simulink model "Copy_of_Single_Phase_SAPF_16apr"  (R2017a)
settings: Solver=ode45  StartTime=0.0  StopTime=10  RelTol=1e-3  EnableMultiTasking=on
libraries: powerlib x23, simulink x1
settings Model: Creator=Niranjan  LastModifiedBy=Dell
settings DataIOCC: LimitDataPoints=on  SaveFormat=Array
settings OptimizationCC: LifeSpan=inf
settings DebuggingCC: SolverPrmCheckMsg=warning  SFUnexpectedBacktrackingDiag=warning  SFNoUnconditionalDefaultTransitionDiag=warning  SFExecutionAtInitializationDiag=none
settings HardwareCC: ProdBitPerPointer=32  ProdBitPerSizeT=32  ProdBitPerPtrDiffT=32  ProdLargestAtomicFloat=None  ProdIntDivRoundTo=Undefined  ProdEndianess=Unspecified  ProdWordSize=32  ProdHWDeviceType=32-bit Generic
settings ModelReferenceCC: PropagateSignalLabelsOutOfModel=off
settings GRTTargetCC: TargetLangStandard=C89/C90 (ANSI)  GeneratePreprocessorConditionals=Disable all
settings ConfigComp: CovMetricSettings=dw  CovHtmlReporting=on  CovSaveCumulativeToWorkspaceVar=on  CovSaveSingleToWorkspaceVar=on  CovExternalEMLEnable=off  CovSFcnEnable=off

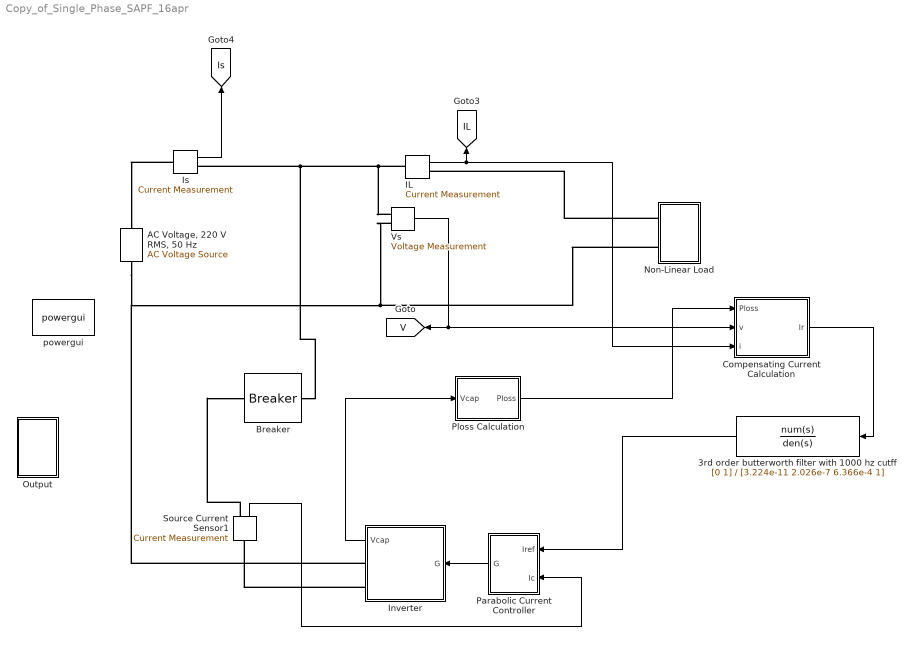
== system Copy_of_Single_Phase_SAPF_16apr ==
  3rd order butterworth filter with 1000 hz cutff : TransferFcn  Numerator=[0 1]  Denominator=[3.224e-11 2.026e-7 6.366e-4 1]
  "AC Voltage, 220 V RMS, 50 Hz" : powerlib/Electrical Sources/AC Voltage Source  Amplitude=311.13  Phase=0  Frequency=50  SampleTime=0  Measurements=None  BusType=swing  Pref=10e3  Qref=0  Qmin=-inf  Qmax=+inf
  Breaker : powerlib/Elements/Breaker  InitialState=0  SwitchingTimes=[0.965]  External=off  BreakerResistance=0.01  SnubberResistance=1e6  SnubberCapacitance=inf  Measurements=None  MoreParameters=on  NoBreakLoop=off
      settings: SourceProductName=Simscape Power Systems
  Compensating Current Calculation : Subsystem
  IL : powerlib/Measurements/Current Measurement  PhasorSimulation=off  OutputType=Complex  PSBequivalent=0
  Inverter : Subsystem
  Is : powerlib/Measurements/Current Measurement  PhasorSimulation=off  OutputType=Complex  PSBequivalent=0
  Non-Linear Load : Subsystem
  Output : Subsystem
  Parabolic Current Controller : Subsystem
  Ploss Calculation : Subsystem
  Source Current Sensor1 : powerlib/Measurements/Current Measurement  PhasorSimulation=off  OutputType=Complex  PSBequivalent=0
  Vs : powerlib/Measurements/Voltage Measurement  PhasorSimulation=off  OutputType=Complex  PSBequivalent=0
  powergui : powerlib/powergui  Priority=1  SimulationMode=Discrete  SampleTime=1e-5  frequency=60  Iterations=50  frequencyindice=50  Pbase=100e6  ErrMax=1e-4  UnitsV=kV  UnitsW=MW  buscounter=0  FunctionMessages=off  echomessages=off  EnableUseOfTLC=off  CurrentSourceSwitches=off  DisableSnubberDevices=off  DisableRonSwitches=off  DisableVfSwitches=off  DisplayEquations=off  SolverType=Tustin/Backward Euler (TBE)  Interpol=off  ExternalGateDelay=off  methode=off  Ts=10  x0status=blocks  SPID=off  SwTol=0  HookPort=off  RestoreLinks=warning  ResistiveCurrentMeasurement=off  Frange=[0:2:500]  Ylog=off  Xlog=on  ShowGrid=off  save=off  variable=ZData  structure=ScopeData_PCC  ZoomFFT=off  StartTime=1.2  cycles=1  DisplayStyle=1  fundamental=50  FreqAxis=on  MaxFrequency=3000  frequencyindicesteady=1  RmsSteady=1  display=off
  tag scope: IL=global, Is=global, V=global
  wires:
  IL/1 -> Compensating Current Calculation/3(i), [IL]
  Vs/1 -> Compensating Current Calculation/2(v), [V]
  Is/1 -> [Is]
  Source Current Sensor1/1 -> Parabolic Current Controller/2(Ic)
  Parabolic Current Controller/1(G) -> Inverter/1(G)
  Inverter/1(Vcap) -> Ploss Calculation/1(Vcap)
  Ploss Calculation/1(Ploss) -> Compensating Current Calculation/1(Ploss)
  Compensating Current Calculation/1(Ir) -> 3rd order butterworth filter with 1000 hz cutff/1
  3rd order butterworth filter with 1000 hz cutff/1 -> Parabolic Current Controller/1(Iref)
  connections:
  Is/LConn1 -- "AC Voltage, 220 V RMS, 50 Hz"/RConn1
  Non-Linear Load/LConn1 -- IL/RConn1
  Inverter/RConn1 -- "AC Voltage, 220 V RMS, 50 Hz"/LConn1 -- Vs/LConn2 -- Non-Linear Load/LConn2
  Inverter/RConn2 -- Source Current Sensor1/LConn1
  IL/LConn1 -- Breaker/RConn1 -- Is/RConn1 -- Vs/LConn1
  Source Current Sensor1/RConn1 -- Breaker/LConn1

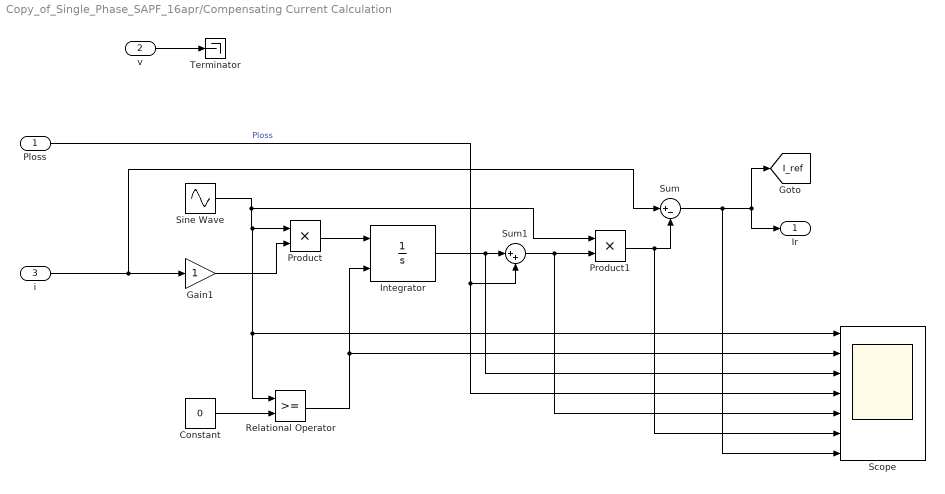
== system Copy_of_Single_Phase_SAPF_16apr/Compensating Current Calculation ==
  Ploss : Inport
  v : Inport  Port=2
  i : Inport  Port=3
  Constant : Constant  Value=0
  Gain1 : Gain
  Integrator : Integrator  ExternalReset=rising
  Product : Product
  Product1 : Product
  Relational Operator : RelationalOperator  OutDataTypeStr=boolean  RndMeth=Simplest
  Scope : Scope  NumInputPorts=7
  Sine Wave : Sin  Frequency=314.16  SampleTime=0
  Sum : Sum  Inputs=|+-
  Sum1 : Sum  Inputs=|++
  Terminator : Terminator
  Ir : Outport
  tag scope: I_ref=global
  wires:
  Gain1/1 -> Product/2
  Sine Wave/1 -> Product/1, Relational Operator/1, Scope/1, Product1/1
  Product/1 -> Integrator/1
  v/1 -> Terminator/1
  Relational Operator/1 -> Integrator/2, Scope/2
  Constant/1 -> Relational Operator/2
  Ploss/1 -> Scope/4, Sum1/2  "Ploss"
  Integrator/1 -> Scope/3, Sum1/1
  Sum1/1 -> Scope/5, Product1/2
  Product1/1 -> Scope/6, Sum/2
  Sum/1 -> Scope/7, Ir/1, [I_ref]
  i/1 -> Sum/1, Gain1/1

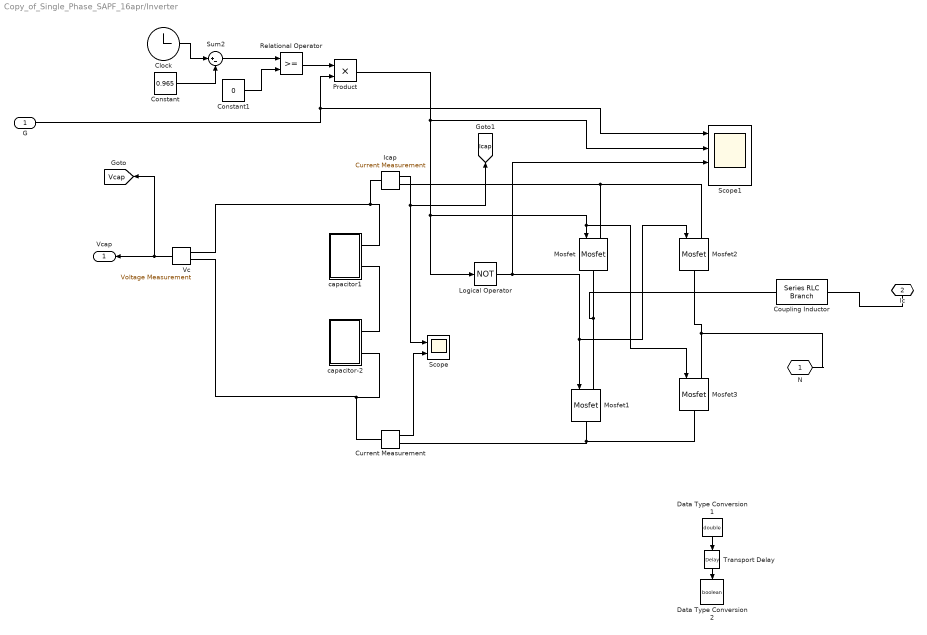
== system Copy_of_Single_Phase_SAPF_16apr/Inverter ==
  G : Inport
  Clock : Clock
  Constant : Constant  Value=0.965
  Constant1 : Constant  Value=0
  Coupling Inductor : powerlib/Elements/Series RLC Branch  LConnTagsString=__new0  RConnTagsString=__new0  BranchType=RL  Resistance=0.12  Inductance=9e-3  SetiL0=off  InitialCurrent=0  Capacitance=0.015  Setx0=off  InitialVoltage=0  Measurements=None
  Current Measurement : powerlib/Measurements/Current Measurement  PhasorSimulation=off  OutputType=Complex  PSBequivalent=0
  Data Type Conversion1 : DataTypeConversion  OutDataTypeStr=double
  Data Type Conversion2 : DataTypeConversion  OutDataTypeStr=boolean
  Icap : powerlib/Measurements/Current Measurement  PhasorSimulation=off  OutputType=Complex  PSBequivalent=0
  Logical Operator : Logic  Operator=NOT  IconShape=distinctive  AllPortsSameDT=off  OutDataTypeStr=boolean
  Mosfet{,1..3} (4 alike) : powerlib/Power Electronics/Mosfet  Ron=0.1  Lon=0  Rd=0.01  Vfd=0  IC=0  Rs=1e5  Cs=inf  Measurements=off
  Product : Product
  Relational Operator : RelationalOperator  OutDataTypeStr=boolean  RndMeth=Simplest
  Scope : Scope  NumInputPorts=2
  Scope1 : Scope  NumInputPorts=4
  Sum2 : Sum  Inputs=|+-
  Transport Delay : TransportDelay  DelayTime=2e-6
  Vc : powerlib/Measurements/Voltage Measurement  PhasorSimulation=off  OutputType=Complex  PSBequivalent=0
  capacitor-2 : Subsystem
  capacitor1 : Subsystem
  N : PMIOPort  Port=1  Side=Right
  Ic : PMIOPort  Port=2  Side=Right
  Vcap : Outport
  tag scope: Icap=global, Vcap=global
  wires:
  Vc/1 -> [Vcap], Vcap/1
  Icap/1 -> Scope/1, [Icap]
  Current Measurement/1 -> Scope/2
  Data Type Conversion1/1 -> Transport Delay/1
  Transport Delay/1 -> Data Type Conversion2/1
  Sum2/1 -> Relational Operator/1
  Clock/1 -> Sum2/1
  Constant/1 -> Sum2/2
  Constant1/1 -> Relational Operator/2
  Relational Operator/1 -> Product/1
  G/1 -> Scope1/1, Product/2
  Logical Operator/1 -> Mosfet2/1, Mosfet1/1, Scope1/3
  Product/1 -> Logical Operator/1, Mosfet3/1, Mosfet/1, Scope1/2
  connections:
  Mosfet1/LConn1 -- Coupling Inductor/RConn1 -- Mosfet/RConn1
  capacitor-2/RConn2 -- Vc/LConn2 -- Current Measurement/LConn1
  Vc/LConn1 -- Icap/LConn1 -- capacitor1/RConn1
  Coupling Inductor/LConn1 -- Ic/RConn1
  Mosfet1/RConn1 -- Mosfet3/RConn1 -- Current Measurement/RConn1
  Mosfet/LConn1 -- Mosfet2/LConn1 -- Icap/RConn1
  capacitor-2/RConn1 -- capacitor1/RConn2
  Mosfet3/LConn1 -- N/RConn1 -- Mosfet2/RConn1

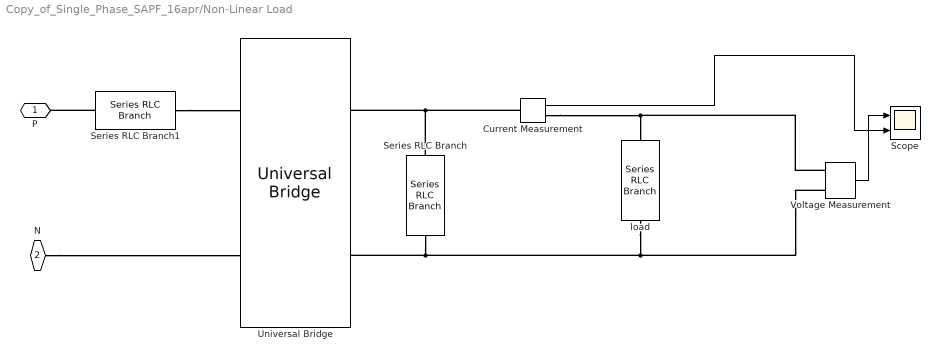
== system Copy_of_Single_Phase_SAPF_16apr/Non-Linear Load ==
  " load" : powerlib/Elements/Series RLC Branch  LConnTagsString=__new0  RConnTagsString=__new0  BranchType=R  Resistance=100  Inductance=1e-3  SetiL0=off  InitialCurrent=0  Capacitance=0.015  Setx0=off  InitialVoltage=0  Measurements=None
  Current Measurement : powerlib/Measurements/Current Measurement  PhasorSimulation=off  OutputType=Complex  PSBequivalent=0
  Scope : Scope  NumInputPorts=2
  Series RLC Branch : powerlib/Elements/Series RLC Branch  LConnTagsString=__new0  RConnTagsString=__new0  BranchType=C  Resistance=1  Inductance=1e-3  SetiL0=off  InitialCurrent=0  Capacitance=3300e-6  Setx0=on  InitialVoltage=235  Measurements=None
  Series RLC Branch1 : powerlib/Elements/Series RLC Branch  LConnTagsString=__new0  RConnTagsString=__new0  BranchType=L  Resistance=1  Inductance=2e-3  SetiL0=off  InitialCurrent=3  Capacitance=1e-6  Setx0=off  InitialVoltage=0  Measurements=None
  Universal Bridge : powerlib/Power Electronics/Universal Bridge  Arms=2  SnubberResistance=1e5  SnubberCapacitance=inf  Device=Diodes  Ron=1e-3  Lon=0  ForwardVoltages="[  0  0  ]"  ForwardVoltage=0  GTOparameters=[ 10e-6 , 20e-6 ]  IGBTparameters=[ 1e-6 , 2e-6 ]  Measurements=None  Measurements_2=None  converterType=Rectifier
  Voltage Measurement : powerlib/Measurements/Voltage Measurement  PhasorSimulation=off  OutputType=Complex  PSBequivalent=0
  P : PMIOPort  Port=1  Side=Left
  N : PMIOPort  Port=2  Side=Left
  wires:
  Voltage Measurement/1 -> Scope/1
  Current Measurement/1 -> Scope/2
  connections:
  Current Measurement/RConn1 -- Voltage Measurement/LConn1 -- " load"/LConn1
  Universal Bridge/RConn2 -- Voltage Measurement/LConn2 -- " load"/RConn1 -- Series RLC Branch/RConn1
  Current Measurement/LConn1 -- Series RLC Branch/LConn1 -- Universal Bridge/RConn1
  N/RConn1 -- Universal Bridge/LConn2
  Series RLC Branch1/RConn1 -- Universal Bridge/LConn1
  Series RLC Branch1/LConn1 -- P/RConn1

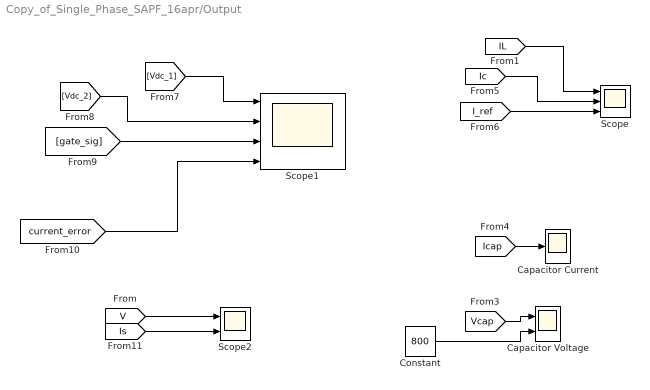
== system Copy_of_Single_Phase_SAPF_16apr/Output ==
  Capacitor Current : Scope
  Capacitor Voltage : Scope  NumInputPorts=2
  Constant : Constant  Value=800
  Scope : Scope  NumInputPorts=3
  Scope1 : Scope  NumInputPorts=4
  Scope2 : Scope  NumInputPorts=2
  wires:
  [Vcap] -> Capacitor Voltage/1
  [Icap] -> Capacitor Current/1
  [I_ref] -> Scope/3
  [IL] -> Scope/1
  Constant/1 -> Capacitor Voltage/2
  [Vdc_1] -> Scope1/1
  [Vdc_2] -> Scope1/2
  [gate_sig] -> Scope1/3
  [current_error] -> Scope1/4
  [Ic] -> Scope/2
  [V] -> Scope2/1
  [Is] -> Scope2/2

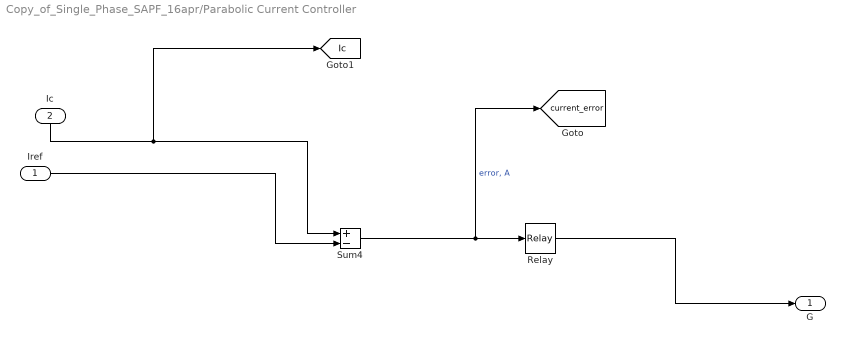
== system Copy_of_Single_Phase_SAPF_16apr/Parabolic Current Controller ==
  Iref : Inport
  Ic : Inport  Port=2
  Relay : Relay  OnSwitchValue=0.5  OffSwitchValue=-0.5
  Sum4 : Sum  Inputs=+-
  G : Outport
  tag scope: Ic=global, current_error=global
  wires:
  Relay/1 -> G/1
  Iref/1 -> Sum4/2
  Ic/1 -> Sum4/1, [Ic]
  Sum4/1 -> Relay/1, [current_error]  "error, A"

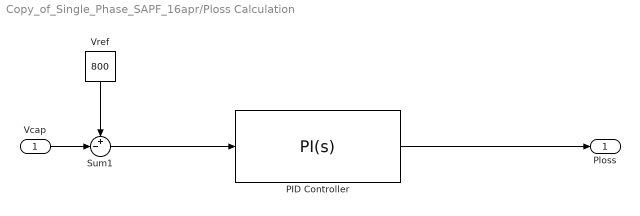
== system Copy_of_Single_Phase_SAPF_16apr/Ploss Calculation ==
  Vcap : Inport
  PID Controller : simulink/Continuous/PID Controller  Controller=PI  TimeDomain=Continuous-time  SampleTime=-1  IntegratorMethod=Forward Euler  FilterMethod=Forward Euler  Form=Parallel  UseFilter=on  ControllerParametersSource=internal  P=800  I=1200  D=0  N=100  InitialConditionSource=internal  InitialConditionForIntegrator=0  InitialConditionForFilter=0  ExternalReset=none  LimitOutput=on  UpperSaturationLimit=1e6  LowerSaturationLimit=-1e6  LinearizeAsGain=on  AntiWindupMode=clamping  Kb=1  TrackingMode=off  Kt=1  PParamMin=[]  PParamMax=[]  IParamMin=[]  IParamMax=[]  DParamMin=[]  DParamMax=[]  NParamMin=[]  NParamMax=[]  KbParamMin=[]  KbParamMax=[]  KtParamMin=[]  KtParamMax=[]  POutMin=[]  POutMax=[]  IOutMin=[]  IOutMax=[]  DOutMin=[]  DOutMax=[]  NOutMin=[]  NOutMax=[]  KbOutMin=[]  KbOutMax=[]  KtOutMin=[]  KtOutMax=[]  IntegratorOutMin=[]  IntegratorOutMax=[]  FilterOutMin=[]  FilterOutMax=[]  SumOutMin=[]  SumOutMax=[]  SumI1OutMin=[]  SumI1OutMax=[]  SumI2OutMin=[]  SumI2OutMax=[]  SumI3OutMin=[]  SumI3OutMax=[]  SumDOutMin=[]  SumDOutMax=[]  SaturationOutMin=[]  SaturationOutMax=[]  IntegratorContinuousStateAttributes=''  IntegratorStateMustResolveToSignalObject=off  IntegratorRTWStateStorageClass=Auto  FilterContinuousStateAttributes=''  FilterStateMustResolveToSignalObject=off  FilterRTWStateStorageClass=Auto  DifferentiatorICPrevScaledInput=0  DifferentiatorOutMin=[]  DifferentiatorOutMax=[]  InitialConditionSetting=State (most efficient)
  Sum1 : Sum  Inputs=+-|
  Vref : Constant  Value=800
  Ploss : Outport
  wires:
  Vcap/1 -> Sum1/2
  Vref/1 -> Sum1/1
  PID Controller/1 -> Ploss/1
  Sum1/1 -> PID Controller/1

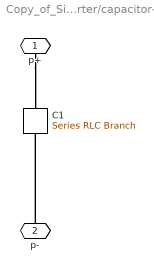
== system Copy_of_Single_Phase_SAPF_16apr/Inverter/capacitor-2 ==
  "C1 " : powerlib/Elements/Series RLC Branch  LConnTagsString=__new0  RConnTagsString=__new0  BranchType=C  Resistance=1e-9  Inductance=1e-9  SetiL0=off  InitialCurrent=0  Capacitance=18000e-6  Setx0=on  InitialVoltage=400  Measurements=None
  p+ : PMIOPort  Port=1  Side=Right
  p- : PMIOPort  Port=2  Side=Right
  connections:
  p-/RConn1 -- "C1 "/RConn1
  p+/RConn1 -- "C1 "/LConn1

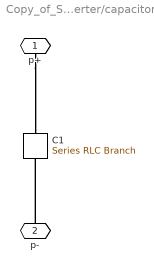
== system Copy_of_Single_Phase_SAPF_16apr/Inverter/capacitor1 ==
  "C1 " : powerlib/Elements/Series RLC Branch  LConnTagsString=__new0  RConnTagsString=__new0  BranchType=C  Resistance=1e-9  Inductance=1e-9  SetiL0=off  InitialCurrent=0  Capacitance=18000e-6  Setx0=on  InitialVoltage=400  Measurements=None
  p+ : PMIOPort  Port=1  Side=Right
  p- : PMIOPort  Port=2  Side=Right
  connections:
  p-/RConn1 -- "C1 "/RConn1
  p+/RConn1 -- "C1 "/LConn1
